simulink model "sampleModel1552_1"  (R2023a)
settings: Solver=VariableStepAuto  StartTime=0.0  StopTime=10.0  RelTol=1e-3
libraries: hdlsllib x5, simulink x3
settings Model: Creator=user1  LastModifiedBy=user1

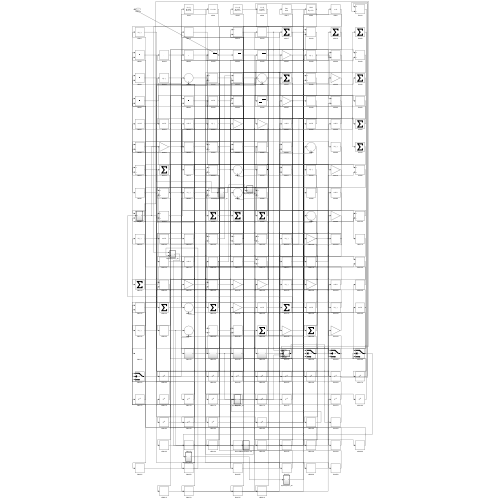
[thumbnail: Simulink's stored preview of the top-level diagram]
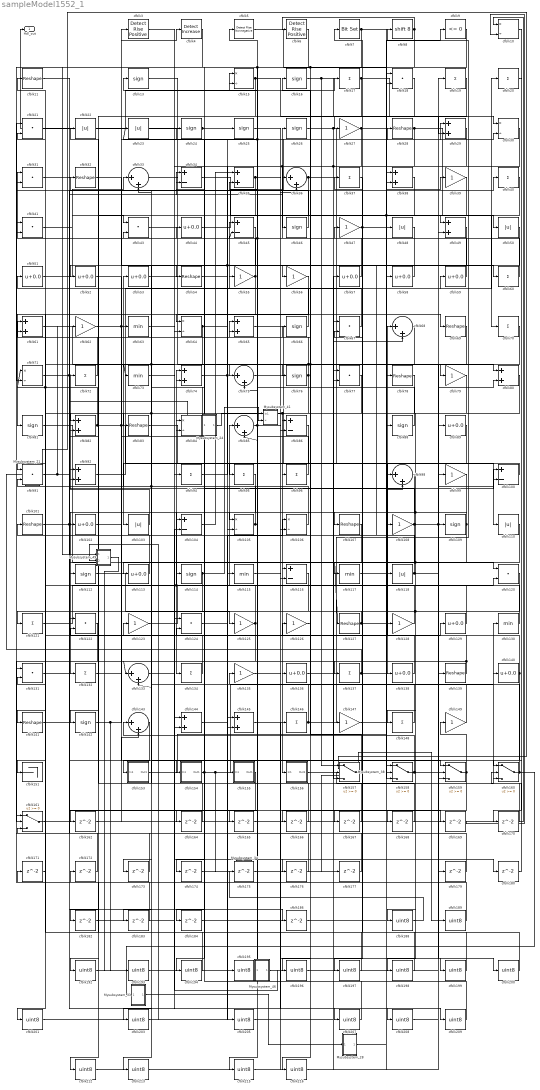
== system sampleModel1552_1 ==
  Mysubsystem_21 : Subsystem  TreatAsAtomicUnit=on  RTWFcnName=Mysubsystem_21
      settings: RTWFcnNameOpts=User specified  RTWFileNameOpts=Use function name
  Mysubsystem_24 : Subsystem  TreatAsAtomicUnit=on  RTWFcnName=Mysubsystem_24
      settings: RTWFcnNameOpts=User specified  RTWFileNameOpts=Use function name
  Mysubsystem_28 : Subsystem  TreatAsAtomicUnit=on  RTWFcnName=Mysubsystem_28
      settings: RTWFcnNameOpts=User specified  RTWFileNameOpts=Use function name
  Mysubsystem_31 : Subsystem  TreatAsAtomicUnit=on  RTWFcnName=Mysubsystem_31
      settings: RTWFcnNameOpts=User specified  RTWFileNameOpts=Use function name
  Mysubsystem_34 : Subsystem  TreatAsAtomicUnit=on  RTWFcnName=Mysubsystem_34
      settings: RTWFcnNameOpts=User specified  RTWFileNameOpts=Use function name
  Mysubsystem_38 : Subsystem  TreatAsAtomicUnit=on  RTWFcnName=Mysubsystem_38
      settings: RTWFcnNameOpts=User specified  RTWFileNameOpts=Use function name
  Mysubsystem_41 : Subsystem  TreatAsAtomicUnit=on  RTWFcnName=Mysubsystem_41
      settings: RTWFcnNameOpts=User specified  RTWFileNameOpts=Use function name
  Mysubsystem_46 : Subsystem  TreatAsAtomicUnit=on  RTWFcnName=Mysubsystem_46
      settings: RTWFcnNameOpts=User specified  RTWFileNameOpts=Use function name
  Mysubsystem_49 : Subsystem  TreatAsAtomicUnit=on  RTWFcnName=Mysubsystem_49
      settings: RTWFcnNameOpts=User specified  RTWFileNameOpts=Use function name
  cfblk{10,15,30,64,71,84,105..106} (8 alike) : Product  Inputs=*/  OutDataTypeStr=uint8  RndMeth=Zero  SaturateOnIntegerOverflow=on
  cfblk{34,45,86,100,104,116} (6 alike) : Sum  Inputs=+-  OutDataTypeStr=uint8
  cfblk{11,28,32,54,69,78,83,101,107,127,139,141} (12 alike) : Reshape
  cfblk{44,51..53,57..59,89,102,113,129,136,138,140} (14 alike) : Bias  Bias=0.0  SaturateOnIntegerOverflow=off
  cfblk{22..23,48,50,103,110,118} (7 alike) : Abs  OutDataTypeStr=uint8  SaturateOnIntegerOverflow=off
  cfblk{27,39,47,55..56,62,79,99,108,123,125..126,128,135,147,149} (16 alike) : Gain  OutDataTypeStr=uint8
  cfblk{13,16,24..26,46,66,76,81,88,109,112,114,142} (14 alike) : Signum
  cfblk{63,73,115,117,130} (5 alike) : MinMax  OutDataTypeStr=uint8
  cfblk{18,21,31,41,43,67,77,91,120,122,124,131} (12 alike) : DotProduct  OutDataTypeStr=uint8
  cfblk{17,19..20,37,40,60,70,72,94..96,121,132,134,137,146,148} (17 alike) : Sum  Inputs=+  OutDataTypeStr=uint8
  cfblk{33,36,68,75,85,98,133,143} (8 alike) : Sum  Inputs=|++  OutDataTypeStr=uint8
  cfblk{29,35,38,49,61,65,74,80,82,92,144..145} (12 alike) : Sum  OutDataTypeStr=uint8
  cfblk151 : Terminator
  cfblk153 : Subsystem
      settings: LibrarySourceBlock=|
      | hdlsllib/Ports &
      | Subsystems/Subsystem
  cfblk154 : Subsystem
      settings: LibrarySourceBlock=|
      | hdlsllib/Ports &
      | Subsystems/Subsystem
  cfblk155 : Subsystem
      settings: LibrarySourceBlock=|
      | hdlsllib/Ports &
      | Subsystems/Subsystem
  cfblk156 : Subsystem
      settings: LibrarySourceBlock=|
      | hdlsllib/Ports &
      | Subsystems/Subsystem
  cfblk{157..161} (5 alike) : Switch  OutDataTypeStr=uint8  SaturateOnIntegerOverflow=off  InputSameDT=off
  cfblk{162,164..177,179..180,182..184,186} (21 alike) : Delay  SampleTime=1
  cfblk{188..189,192..201,203,205,207..209,212..213,215..216} (21 alike) : DataTypeConversion  OutDataTypeStr=uint8  SaturateOnIntegerOverflow=off  RndMeth=Floor
  cfblk3 : hdlsllib/Logic and Bit Operations/Detect Rise Positive  vinit=0  OutDataTypeStr=uint8
  cfblk4 : simulink/Logic and Bit Operations/Detect Increase  vinit=0.0  OutDataTypeStr=uint8
      settings: LibrarySourceBlock=|
      | hdlsllib/Logic and Bit
      | Operations/Detect
      | Increase
  cfblk5 : hdlsllib/Logic and Bit Operations/Detect Rise Nonnegative  vinit=0  OutDataTypeStr=uint8
  cfblk6 : hdlsllib/Logic and Bit Operations/Detect Rise Positive  vinit=0  OutDataTypeStr=uint8
  cfblk7 : simulink/Logic and Bit Operations/Bit Set  iBit=0
      settings: LibrarySourceBlock=|
      | hdlsllib/Logic and Bit
      | Operations/Bit Set
  cfblk8 : ArithShift  BitShiftNumber=8
  cfblk9 : hdlsllib/Logic and Bit Operations/Compare To Zero  relop=<=  OutDataTypeStr=uint8
  Hdl_out : Outport  OutDataTypeStr=uint8
  wires:
  cfblk104/1 -> cfblk35/1
  cfblk44/1 -> cfblk29/1
  cfblk48/1 -> cfblk101/1
  cfblk158/1 -> cfblk143/1, cfblk80/2
  cfblk146/1 -> cfblk8/1, cfblk34/1
  cfblk106/1 -> cfblk53/1
  cfblk156/1(Out1) -> cfblk130/1
  cfblk84/1 -> cfblk32/1
  cfblk130/1 -> cfblk74/1, cfblk91/2
  cfblk17/1 -> cfblk30/1, cfblk86/1
  cfblk154/1(Out1) -> cfblk140/1, cfblk175/1, cfblk174/1
  cfblk103/1 -> cfblk72/1
  cfblk112/1 -> cfblk125/1
  cfblk56/1 -> cfblk81/1
  cfblk98/1 -> cfblk132/1
  cfblk140/1 -> cfblk68/1, cfblk173/1
  cfblk96/1 -> cfblk13/1, cfblk23/1, cfblk45/2
  cfblk81/1 -> cfblk120/1
  cfblk36/1 -> cfblk49/1, cfblk64/2
  cfblk92/1 -> cfblk45/1
  cfblk64/1 -> cfblk76/1, cfblk203/1
  cfblk95/1 -> cfblk134/1
  cfblk77/1 -> cfblk156/1(In1), cfblk154/1(In1)
  cfblk116/1 -> cfblk136/1
  cfblk88/1 -> cfblk51/1
  cfblk113/1 -> cfblk22/1
  cfblk61/1 -> cfblk94/1
  cfblk82/1 -> cfblk96/1, cfblk28/1, cfblk61/1
  cfblk114/1 -> Mysubsystem_41/2(u), cfblk142/1
  cfblk108/1 -> cfblk100/2, cfblk200/1, cfblk118/1, cfblk84/2
  cfblk15/1 -> cfblk102/1, cfblk27/1
  cfblk126/1 -> cfblk16/1
  cfblk27/1 -> cfblk77/2, cfblk165/1, cfblk98/2
  cfblk51/1 -> cfblk33/1
  cfblk53/1 -> cfblk75/1
  cfblk133/1 -> cfblk120/2
  cfblk58/1 -> cfblk52/1
  cfblk13/1 -> cfblk109/1
  cfblk101/1 -> cfblk100/1, cfblk186/1
  cfblk57/1 -> cfblk26/1
  cfblk141/1 -> cfblk129/1
  cfblk78/1 -> cfblk82/1
  cfblk46/1 -> cfblk31/1
  cfblk30/1 -> cfblk46/1, cfblk105/2, cfblk157/3
  cfblk26/1 -> cfblk138/1, cfblk60/1
  cfblk6/1 -> cfblk104/1
  cfblk28/1 -> cfblk50/1, cfblk184/1
  cfblk70/1 -> cfblk196/1, cfblk201/1
  cfblk35/1 -> cfblk112/1, cfblk36/2
  cfblk23/1 -> cfblk69/1
  cfblk45/1 -> cfblk54/1
  cfblk22/1 -> cfblk17/1
  cfblk33/1 -> cfblk78/1
  cfblk89/1 -> cfblk137/1
  cfblk10/1 -> cfblk160/1
  cfblk60/1 -> cfblk7/1
  cfblk118/1 -> cfblk89/1, cfblk47/1
  cfblk63/1 -> cfblk144/1
  cfblk76/1 -> cfblk73/1, cfblk61/2, cfblk91/1
  cfblk109/1 -> cfblk127/1, cfblk148/1, cfblk105/1
  cfblk149/1 -> cfblk126/1
  cfblk52/1 -> cfblk159/1
  cfblk128/1 -> cfblk114/1
  cfblk41/1 -> cfblk43/1
  cfblk121/1 -> cfblk85/1
  cfblk147/1 -> cfblk108/1
  cfblk117/1 -> cfblk58/1
  cfblk129/1 -> cfblk5/1
  cfblk137/1 -> Mysubsystem_21/1(In1), cfblk9/1
  cfblk55/1 -> cfblk31/2, cfblk151/1
  cfblk67/1 -> cfblk24/1
  cfblk161/1 -> cfblk10/1
  cfblk139/1 -> cfblk71/1, cfblk41/2, cfblk133/1
  cfblk5/1 -> cfblk158/1
  cfblk86/1 -> cfblk103/1
  cfblk49/1 -> cfblk113/1
  cfblk159/1 -> cfblk149/1, cfblk216/1
  cfblk47/1 -> cfblk117/1, cfblk80/1
  cfblk34/1 -> cfblk70/1
  cfblk65/1 -> cfblk139/1
  cfblk9/1 -> cfblk85/2, cfblk64/1, cfblk116/1
  cfblk16/1 -> cfblk29/2, cfblk157/1
  cfblk31/1 -> cfblk159/2
  cfblk79/1 -> cfblk128/1
  cfblk122/1 -> cfblk141/1
  cfblk25/1 -> cfblk79/1
  cfblk62/1 -> cfblk20/1, cfblk34/2
  cfblk75/1 -> cfblk110/1
  cfblk69/1 -> cfblk83/1, cfblk182/1
  cfblk72/1 -> cfblk11/1
  cfblk157/1 -> cfblk66/1
  cfblk123/1 -> cfblk98/1
  cfblk148/1 -> cfblk92/1
  cfblk131/1 -> cfblk40/1
  cfblk24/1 -> cfblk25/1, Hdl_out/1
  cfblk136/1 -> cfblk68/2
  cfblk100/1 -> cfblk95/1
  cfblk94/1 -> cfblk30/2
  cfblk127/1 -> cfblk121/1, cfblk39/1
  cfblk134/1 -> cfblk123/1
  cfblk80/1 -> cfblk92/2, cfblk133/2
  cfblk138/1 -> cfblk122/2
  cfblk40/1 -> cfblk107/1, cfblk158/3
  cfblk144/1 -> cfblk106/1
  cfblk120/1 -> cfblk162/1, cfblk188/1
  cfblk153/1(Out1) -> cfblk88/1
  cfblk32/1 -> cfblk56/1
  cfblk102/1 -> cfblk84/1
  cfblk29/1 -> cfblk144/2
  cfblk99/1 -> cfblk157/2, cfblk198/1
  cfblk8/1 -> cfblk6/1, cfblk71/2
  cfblk43/1 -> cfblk116/2, cfblk115/1
  cfblk66/1 -> cfblk15/1
  cfblk132/1 -> cfblk3/1
  cfblk59/1 -> cfblk43/2
  cfblk39/1 -> cfblk106/2
  cfblk125/1 -> cfblk161/2, cfblk44/1
  cfblk91/1 -> cfblk62/1, cfblk169/1
  cfblk7/1 -> cfblk159/3, cfblk75/2
  cfblk142/1 -> cfblk4/1, cfblk193/1
  cfblk85/1 -> cfblk65/1, cfblk180/1
  cfblk71/1 -> Mysubsystem_24/1(In1), cfblk36/1
  cfblk105/1 -> cfblk41/1, cfblk63/1, cfblk55/1
  cfblk83/1 -> cfblk147/1
  cfblk74/1 -> cfblk59/1, cfblk86/2
  cfblk143/1 -> cfblk153/1(In1)
  cfblk160/1 -> Mysubsystem_31/1(In1), cfblk67/2
  cfblk162/1 -> cfblk143/2
  cfblk110/1 -> cfblk164/1
  cfblk164/1 -> cfblk33/2
  cfblk165/1 -> cfblk49/2
  cfblk68/1 -> cfblk166/1
  cfblk166/1 -> cfblk35/2
  cfblk115/1 -> cfblk167/1
  cfblk167/1 -> cfblk74/2
  cfblk11/1 -> cfblk168/1
  cfblk168/1 -> cfblk82/2
  cfblk169/1 -> cfblk10/2
  cfblk20/1 -> cfblk170/1
  cfblk170/1 -> cfblk160/2
  cfblk171/1 -> cfblk131/2
  cfblk172/1 -> cfblk21/1
  cfblk173/1 -> cfblk161/3
  cfblk174/1 -> cfblk77/1
  cfblk175/1 -> cfblk15/2
  cfblk3/1 -> cfblk176/1
  cfblk176/1 -> cfblk65/2
  cfblk177/1 -> cfblk122/1
  cfblk179/1 -> cfblk67/1
  cfblk180/1 -> cfblk160/3
  cfblk182/1 -> cfblk104/2
  cfblk50/1 -> cfblk183/1
  cfblk183/1 -> cfblk161/1
  cfblk184/1 -> cfblk158/2
  cfblk186/1 -> cfblk48/1
  cfblk189/1 -> cfblk131/1
  cfblk155/1(Out1) -> cfblk192/1
  cfblk192/1 -> cfblk99/1
  cfblk193/1 -> cfblk155/1(In1)
  cfblk38/1 -> cfblk194/1
  cfblk194/1 -> cfblk172/1
  cfblk54/1 -> cfblk195/1
  cfblk195/1 -> cfblk38/1
  cfblk196/1 -> cfblk38/2
  cfblk37/1 -> cfblk197/1
  cfblk197/1 -> cfblk21/2
  cfblk198/1 -> cfblk37/1
  cfblk145/1 -> cfblk199/1
  cfblk199/1 -> cfblk171/1
  cfblk200/1 -> cfblk145/1
  cfblk201/1 -> cfblk145/2
  cfblk124/1 -> cfblk205/1
  cfblk205/1 -> cfblk57/1
  cfblk21/1 -> cfblk207/1
  cfblk207/1 -> cfblk124/2
  cfblk135/1 -> cfblk208/1
  cfblk208/1 -> cfblk179/1
  cfblk73/1 -> cfblk209/1
  cfblk209/1 -> cfblk135/1
  cfblk18/1 -> cfblk212/1
  cfblk212/1 -> cfblk146/1
  cfblk107/1 -> cfblk213/1
  cfblk213/1 -> cfblk18/1
  cfblk19/1 -> cfblk215/1
  cfblk215/1 -> cfblk177/1
  cfblk216/1 -> cfblk19/1
  Mysubsystem_28/1(Out1) -> cfblk18/2
  Mysubsystem_31/1(Out1) -> Mysubsystem_28/1(In1)
  cfblk188/1 -> Mysubsystem_34/1(In1)
  Mysubsystem_21/1(Y) -> Mysubsystem_38/1(In1)
  Mysubsystem_34/1(Out1) -> Mysubsystem_38/2(In2)
  Mysubsystem_38/1(Out1) -> cfblk189/1
  Mysubsystem_24/1(Out1) -> Mysubsystem_41/1(In1)
  Mysubsystem_46/1(Out1) -> cfblk124/1
  cfblk4/1 -> Mysubsystem_49/1(In1)
  cfblk203/1 -> Mysubsystem_49/2(In2)
  Mysubsystem_49/1(Out1) -> Mysubsystem_46/1(In1)

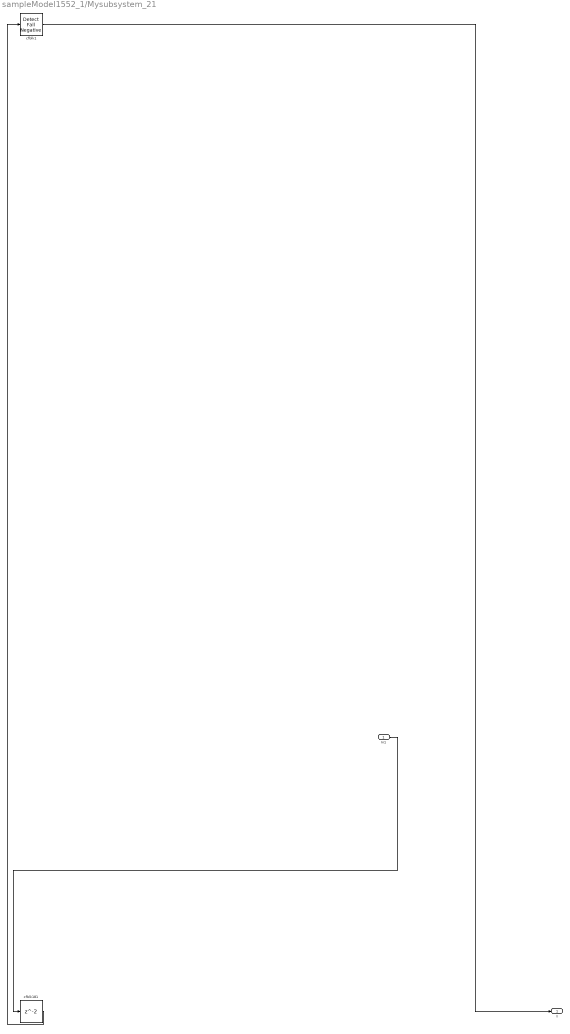
== system sampleModel1552_1/Mysubsystem_21 ==
  In1 : Inport
  cfblk1 : hdlsllib/Logic and Bit Operations/Detect Fall Negative  vinit=0  OutDataTypeStr=boolean
  cfblk181 : Delay  SampleTime=1
  Y : Outport
  wires:
  cfblk181/1 -> cfblk1/1
  In1/1 -> cfblk181/1
  cfblk1/1 -> Y/1

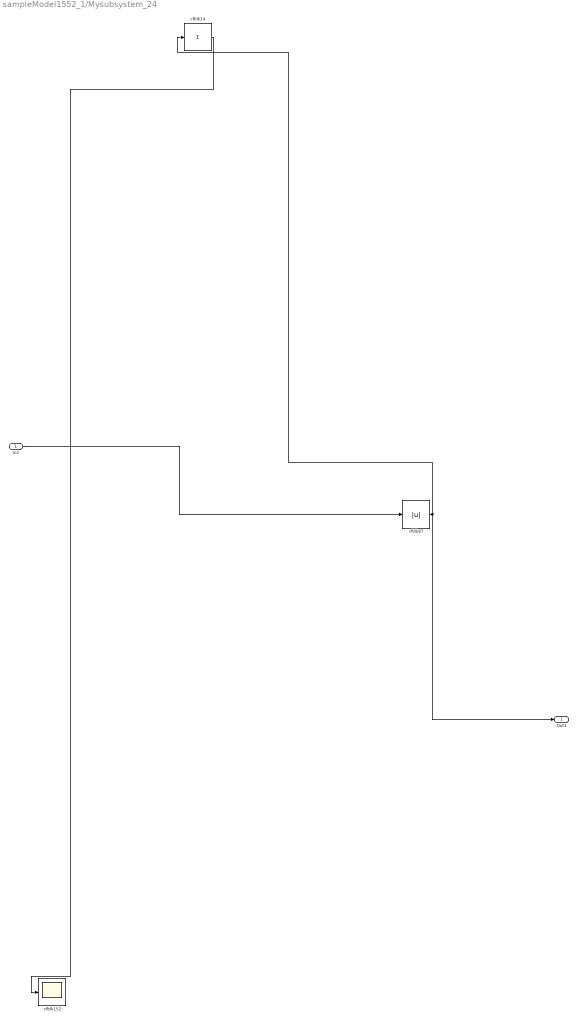
== system sampleModel1552_1/Mysubsystem_24 ==
  In1 : Inport
  cfblk14 : Sum  Inputs=+
  cfblk152 : Scope
  cfblk87 : Abs  SaturateOnIntegerOverflow=off
  Out1 : Outport
  wires:
  cfblk87/1 -> Out1/1, cfblk14/1
  In1/1 -> cfblk87/1
  cfblk14/1 -> cfblk152/1

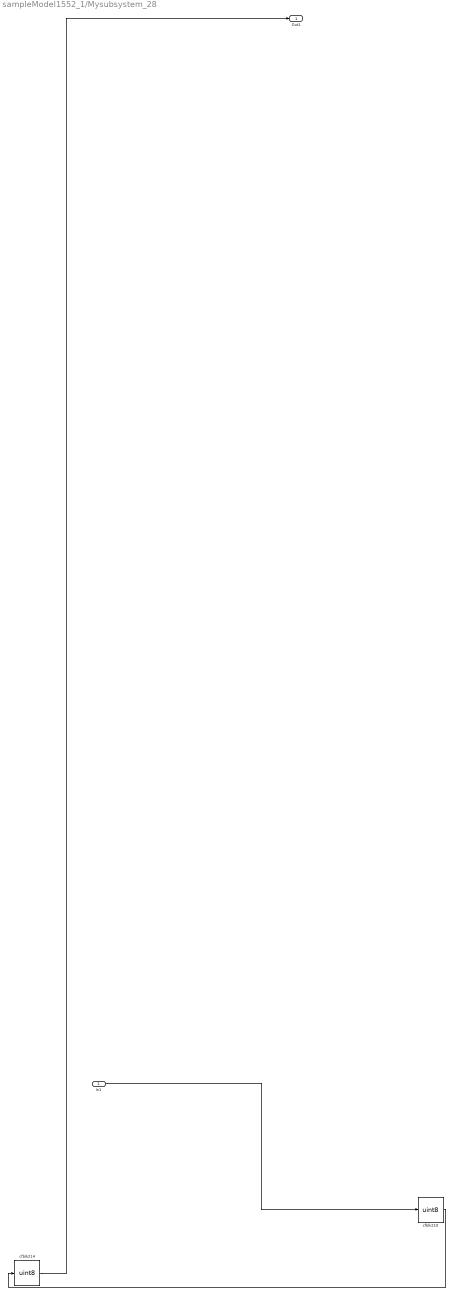
== system sampleModel1552_1/Mysubsystem_28 ==
  In1 : Inport
  cfblk210 : DataTypeConversion  OutDataTypeStr=uint8  SaturateOnIntegerOverflow=off  RndMeth=Floor
  cfblk214 : DataTypeConversion  OutDataTypeStr=uint8  SaturateOnIntegerOverflow=off  RndMeth=Floor
  Out1 : Outport
  wires:
  cfblk210/1 -> cfblk214/1
  In1/1 -> cfblk210/1
  cfblk214/1 -> Out1/1

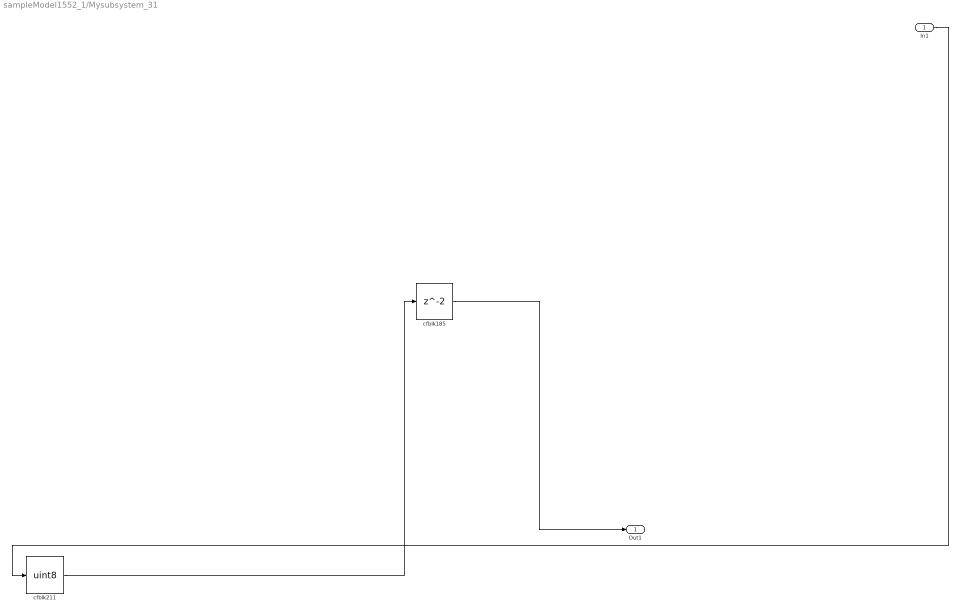
== system sampleModel1552_1/Mysubsystem_31 ==
  In1 : Inport
  cfblk185 : Delay  SampleTime=1
  cfblk211 : DataTypeConversion  OutDataTypeStr=uint8  SaturateOnIntegerOverflow=off  RndMeth=Floor
  Out1 : Outport
  wires:
  cfblk211/1 -> cfblk185/1
  In1/1 -> cfblk211/1
  cfblk185/1 -> Out1/1

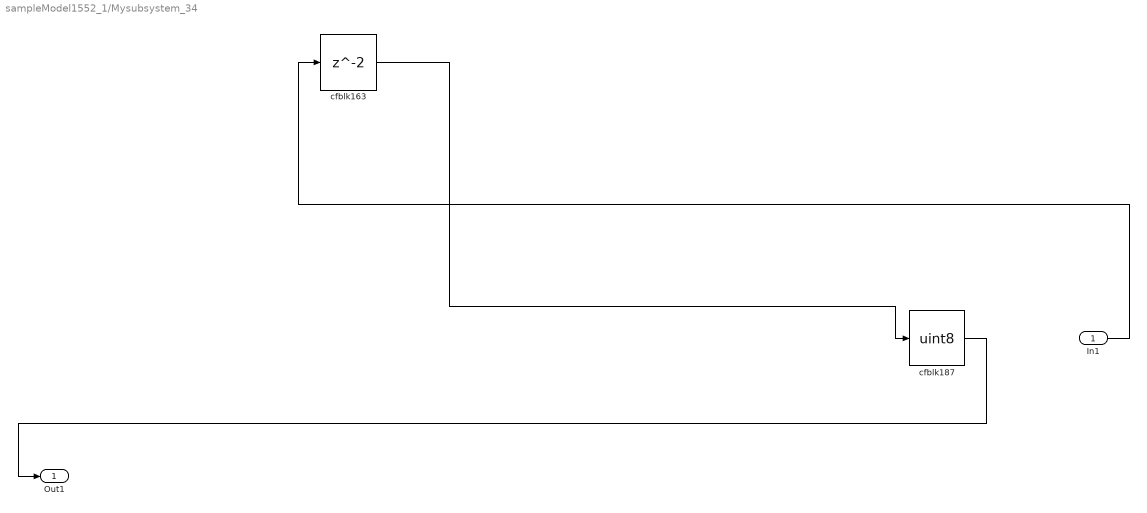
== system sampleModel1552_1/Mysubsystem_34 ==
  In1 : Inport
  cfblk163 : Delay  SampleTime=1
  cfblk187 : DataTypeConversion  OutDataTypeStr=uint8  SaturateOnIntegerOverflow=off  RndMeth=Floor
  Out1 : Outport
  wires:
  cfblk163/1 -> cfblk187/1
  cfblk187/1 -> Out1/1
  In1/1 -> cfblk163/1

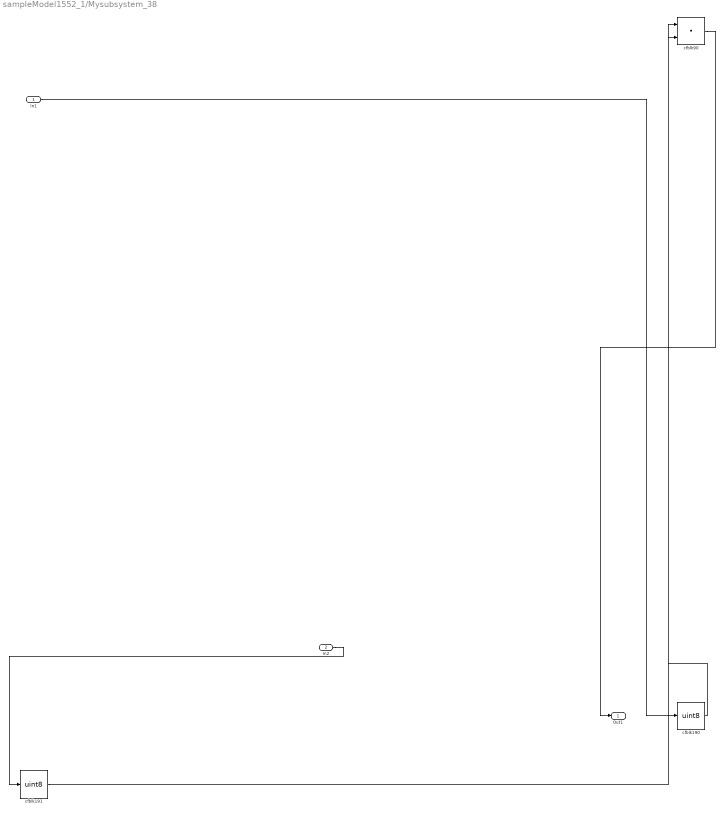
== system sampleModel1552_1/Mysubsystem_38 ==
  In1 : Inport
  In2 : Inport  Port=2
  cfblk190 : DataTypeConversion  OutDataTypeStr=uint8  SaturateOnIntegerOverflow=off  RndMeth=Floor
  cfblk191 : DataTypeConversion  OutDataTypeStr=uint8  SaturateOnIntegerOverflow=off  RndMeth=Floor
  cfblk90 : DotProduct  OutDataTypeStr=Inherit: Inherit via internal rule
  Out1 : Outport
  wires:
  cfblk191/1 -> cfblk90/2
  cfblk190/1 -> cfblk90/1
  cfblk90/1 -> Out1/1
  In1/1 -> cfblk190/1
  In2/1 -> cfblk191/1

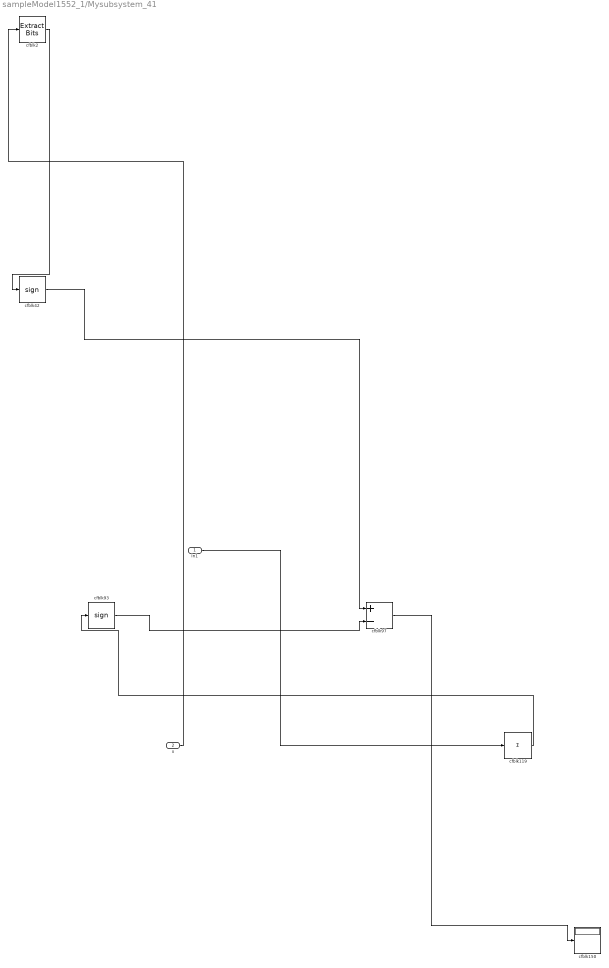
== system sampleModel1552_1/Mysubsystem_41 ==
  In1 : Inport
  u : Inport  Port=2
  cfblk119 : Sum  Inputs=+
  cfblk150 : Display
  cfblk2 : simulink/Logic and Bit Operations/Extract Bits  bitsToExtract=Upper half  numBits=8  bitIdxRange=[0 7]  outScalingMode=Preserve fixed-point scaling
      settings: LibrarySourceBlock=|
      | hdlsllib/Logic and Bit
      | Operations/Extract Bits
  cfblk42 : Signum
  cfblk93 : Signum
  cfblk97 : Sum  Inputs=+-
  wires:
  cfblk119/1 -> cfblk93/1
  cfblk97/1 -> cfblk150/1
  In1/1 -> cfblk119/1
  cfblk93/1 -> cfblk97/2
  cfblk42/1 -> cfblk97/1
  u/1 -> cfblk2/1
  cfblk2/1 -> cfblk42/1

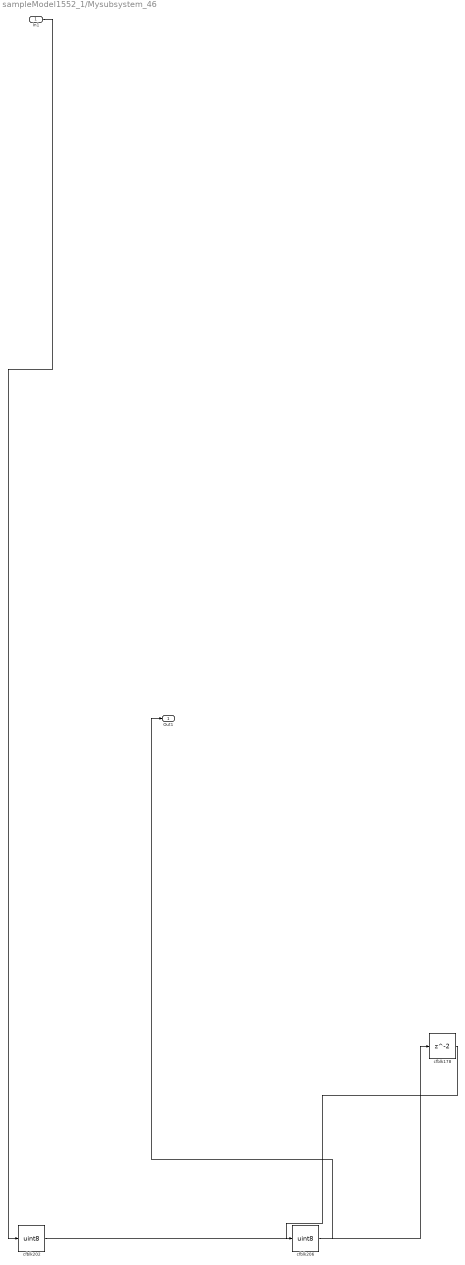
== system sampleModel1552_1/Mysubsystem_46 ==
  In1 : Inport
  cfblk178 : Delay  SampleTime=1
  cfblk202 : DataTypeConversion  OutDataTypeStr=uint8  SaturateOnIntegerOverflow=off  RndMeth=Floor
  cfblk206 : DataTypeConversion  OutDataTypeStr=uint8  SaturateOnIntegerOverflow=off  RndMeth=Floor
  Out1 : Outport
  wires:
  cfblk202/1 -> cfblk178/1
  In1/1 -> cfblk202/1
  cfblk178/1 -> cfblk206/1
  cfblk206/1 -> Out1/1

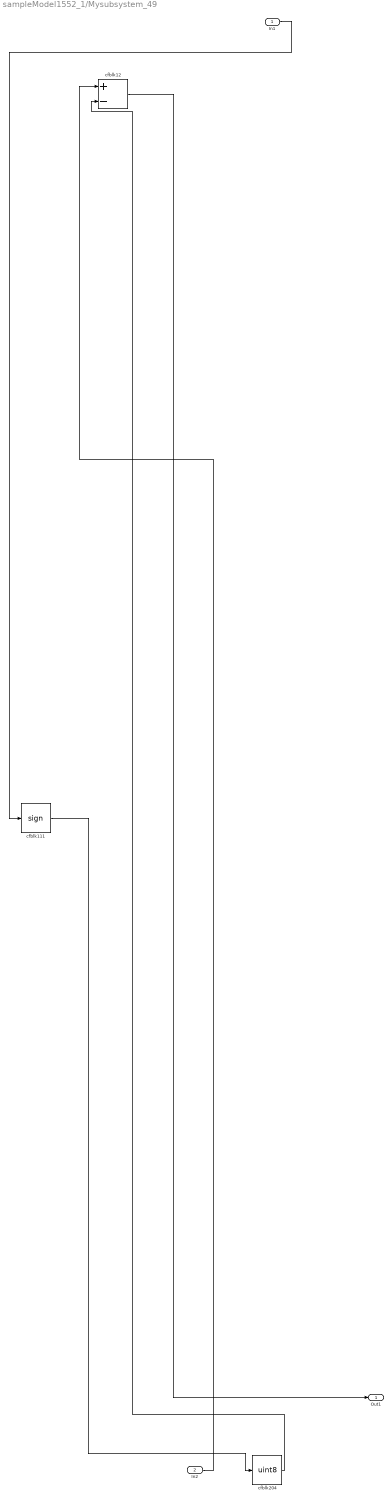
== system sampleModel1552_1/Mysubsystem_49 ==
  In1 : Inport
  In2 : Inport  Port=2
  cfblk111 : Signum
  cfblk12 : Sum  Inputs=+-
  cfblk204 : DataTypeConversion  OutDataTypeStr=uint8  SaturateOnIntegerOverflow=off  RndMeth=Floor
  Out1 : Outport
  wires:
  In1/1 -> cfblk111/1
  cfblk111/1 -> cfblk204/1
  cfblk204/1 -> cfblk12/2
  In2/1 -> cfblk12/1
  cfblk12/1 -> Out1/1

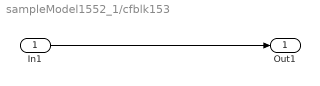
== system sampleModel1552_1/cfblk153 ==
  In1 : Inport
  Out1 : Outport
  wires:
  In1/1 -> Out1/1

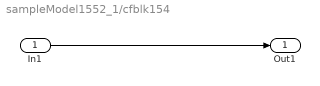
== system sampleModel1552_1/cfblk154 ==
  In1 : Inport
  Out1 : Outport
  wires:
  In1/1 -> Out1/1

== system sampleModel1552_1/cfblk155 ==
  In1 : Inport
  Out1 : Outport
  wires:
  In1/1 -> Out1/1

== system sampleModel1552_1/cfblk156 ==
  In1 : Inport
  Out1 : Outport
  wires:
  In1/1 -> Out1/1
